simulink model "signal_control_system"  (R2023a)
settings: Solver=FixedStepDiscrete  StartTime=0.0  StopTime=20  FixedStep=1  RelTol=1e-3
settings Model: Creator=Administrator  LastModifiedBy=Administrator
settings DataIOCC: ExternalInput=[t, ia, ib, ic, Tlevel, PClimit, set_val, PC, FC]  LoadExternalInput=on  SaveFormat=Structure  ReturnWorkspaceOutputs=off

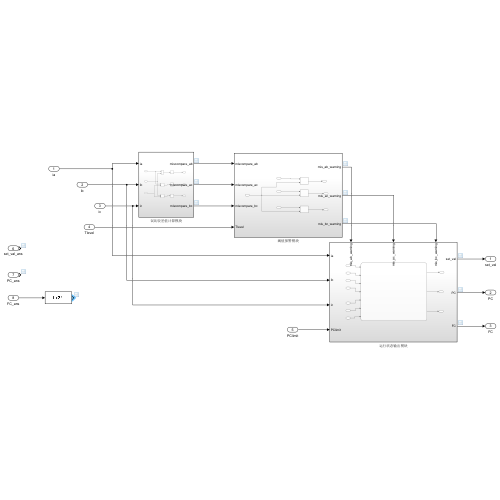
[thumbnail: Simulink's stored preview of the top-level diagram]
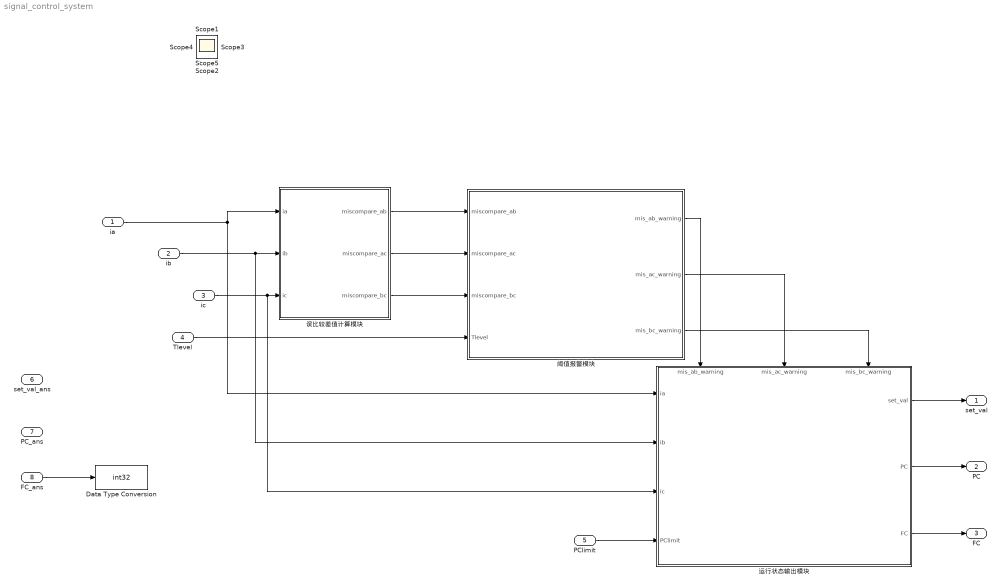
== system signal_control_system ==
  ia : Inport  PortDimensions=1
  ib : Inport  Port=2  PortDimensions=1
  ic : Inport  Port=3  PortDimensions=1
  Tlevel : Inport  Port=4  PortDimensions=1
  PClimit : Inport  Port=5  OutDataTypeStr=double  PortDimensions=1
  set_val_ans : Inport  Port=6
  PC_ans : Inport  Port=7
  FC_ans : Inport  Port=8  OutDataTypeStr=double
  Data Type Conversion : DataTypeConversion  OutDataTypeStr=int32  SaturateOnIntegerOverflow=off  RndMeth=Floor
  误比较差值计算模块 : Subsystem
  运行状态输出模块 : Subsystem
      settings: PortSchema="{\"entries\":[{\"content\":{\"sides\":[{\"content\":{\"connectorIds\":[\"In1\",\"In2\",\"In3\",\"In4\"]},\"type\":\"ConnectorPlacement.EquallySpacedRectSide\",\"uuid\":\"c2265341-80b0-436b-af31-29986e0e6bdd\"},{\"content\":{\"connectorIds\":[\"Out1\",\"Out2\",\"Out3\"],\"side\":\"RIGHT\"},\"type\":\"ConnectorPlacement.EquallySpacedRectSide\",\"uuid\":\"b242c194-baa4-408e-b219-ab790b6c0c89\"},{\"content\":{\"connectorIds\":[\"In5\",\"In6\",\"In7\"],\"side\":\"TOP\"},\"type\":\"ConnectorPlacement.EquallySpacedRectSide\",\"uuid\":\"72118fcd-d084-4d5a-ad77-022196fa3641\"}]},\"type\":\"ConnectorPlacement.EquallySpacedConnector\",\"uuid\":\"1dca4bdc-c94a-404e-99f4-c038544fbae3\"}],\"packageUris\":[\"http://schema.mathworks.com/mf0/Connector/R2020b\"],\"version\":\"1.0\"}"
  阈值报警模块 : Subsystem
  set_val : Outport
  PC : Outport  Port=2
  FC : Outport  Port=3
  Scope{,1..5} (6 alike) : Scope
  wires:
  ia/1 -> 运行状态输出模块/1(ia), 误比较差值计算模块/1(ia)
  ib/1 -> 运行状态输出模块/2(ib), 误比较差值计算模块/2(ib)
  ic/1 -> 误比较差值计算模块/3(ic), 运行状态输出模块/3(ic)
  误比较差值计算模块/1(miscompare_ab) -> 阈值报警模块/1(miscompare_ab)
  误比较差值计算模块/2(miscompare_ac) -> 阈值报警模块/2(miscompare_ac)
  误比较差值计算模块/3(miscompare_bc) -> 阈值报警模块/3(miscompare_bc)
  Tlevel/1 -> 阈值报警模块/4(Tlevel)
  阈值报警模块/1(mis_ab_warning) -> 运行状态输出模块/5(mis_ab_warning)
  阈值报警模块/2(mis_ac_warning) -> 运行状态输出模块/6(mis_ac_warning)
  阈值报警模块/3(mis_bc_warning) -> 运行状态输出模块/7(mis_bc_warning)
  运行状态输出模块/1(set_val) -> set_val/1
  运行状态输出模块/2(PC) -> PC/1
  运行状态输出模块/3(FC) -> FC/1
  PClimit/1 -> 运行状态输出模块/4(PClimit)
  FC_ans/1 -> Data Type Conversion/1

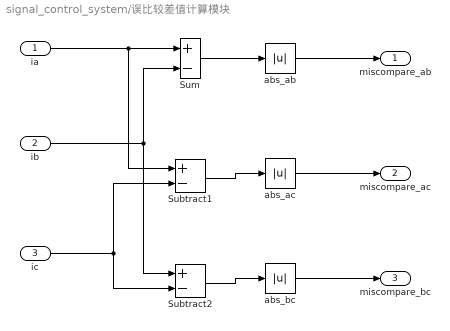
== system signal_control_system/误比较差值计算模块 ==
  ia : Inport
  ib : Inport  Port=2
  ic : Inport  Port=3
  Subtract1 : Sum  Inputs=+-
  Subtract2 : Sum  Inputs=+-
  Sum : Sum  Inputs=+-
  abs_ab : Abs  SaturateOnIntegerOverflow=off
  abs_ac : Abs  SaturateOnIntegerOverflow=off
  abs_bc : Abs  SaturateOnIntegerOverflow=off
  miscompare_ab : Outport
  miscompare_ac : Outport  Port=2
  miscompare_bc : Outport  Port=3
  wires:
  ia/1 -> Subtract1/1, Sum/1
  Subtract1/1 -> abs_ac/1
  abs_bc/1 -> miscompare_bc/1
  abs_ac/1 -> miscompare_ac/1
  Sum/1 -> abs_ab/1
  Subtract2/1 -> abs_bc/1
  abs_ab/1 -> miscompare_ab/1
  ic/1 -> Subtract2/2, Subtract1/2
  ib/1 -> Sum/2, Subtract2/1

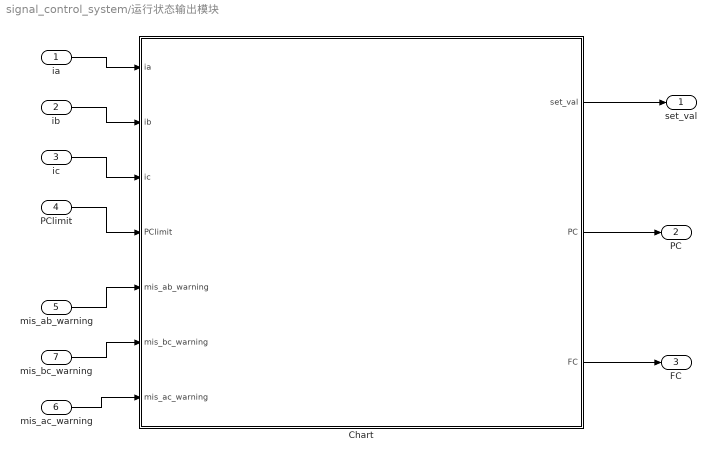
== system signal_control_system/运行状态输出模块 ==
  ia : Inport
  ib : Inport  Port=2
  ic : Inport  Port=3
  PClimit : Inport  Port=4
  mis_ab_warning : Inport  Port=5  OutDataTypeStr=boolean
  mis_ac_warning : Inport  Port=6  OutDataTypeStr=boolean
  mis_bc_warning : Inport  Port=7  OutDataTypeStr=boolean
  Chart : Stateflow chart  TreatAsAtomicUnit=on
  set_val : Outport
  PC : Outport  Port=2
  FC : Outport  Port=3
  wires:
  ia/1 -> Chart/1(ia)
  ib/1 -> Chart/2(ib)
  ic/1 -> Chart/3(ic)
  PClimit/1 -> Chart/4(PClimit)
  mis_ab_warning/1 -> Chart/5(mis_ab_warning)
  mis_bc_warning/1 -> Chart/6(mis_bc_warning)
  mis_ac_warning/1 -> Chart/7(mis_ac_warning)
  Chart/1(set_val) -> set_val/1
  Chart/2(PC) -> PC/1
  Chart/3(FC) -> FC/1

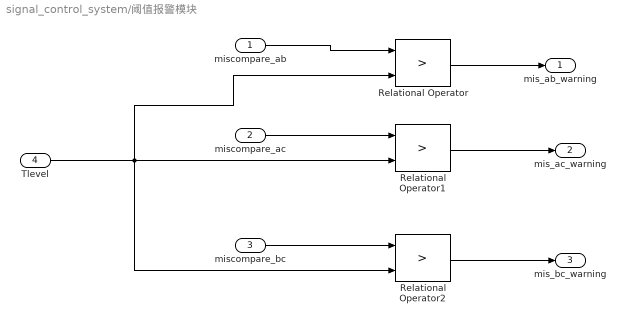
== system signal_control_system/阈值报警模块 ==
  miscompare_ab : Inport
  miscompare_ac : Inport  Port=2
  miscompare_bc : Inport  Port=3
  Tlevel : Inport  Port=4
  Relational Operator : RelationalOperator  Operator=>  OutDataTypeStr=boolean  RndMeth=Simplest
  Relational Operator1 : RelationalOperator  Operator=>  OutDataTypeStr=boolean  RndMeth=Simplest
  Relational Operator2 : RelationalOperator  Operator=>  OutDataTypeStr=boolean  RndMeth=Simplest
  mis_ab_warning : Outport  OutDataTypeStr=boolean
  mis_ac_warning : Outport  Port=2  OutDataTypeStr=boolean
  mis_bc_warning : Outport  Port=3  OutDataTypeStr=boolean
  wires:
  Tlevel/1 -> Relational Operator/2, Relational Operator2/2, Relational Operator1/2
  Relational Operator1/1 -> mis_ac_warning/1
  miscompare_ac/1 -> Relational Operator1/1
  Relational Operator2/1 -> mis_bc_warning/1
  Relational Operator/1 -> mis_ab_warning/1
  miscompare_ab/1 -> Relational Operator/1
  miscompare_bc/1 -> Relational Operator2/1

== stateflow chart signal_control_system/运行状态输出模块/Chart ==
  state SingleFault_ia
    entry:
    FC = 1;
    PC = 0;
    set_val = (ib + ic) / 2;
    during:
    set_val = (ib + ic) / 2;
    if (mis_ab_warning && mis_ac_warning && mis_bc_warning)
    PC = PC + 1;
    end
  state NoFault
    entry:
    FC = 0;
    PC = 0;
    set_val  = median([ia, ib, ic]);
    during:
    set_val  = median([ia, ib, ic]);
    if (~mis_ab_warning && ~mis_ac_warning && ~mis_bc_warning)
    PC = PC ;
    else
    PC = PC + 1;
    end
  state MultiFault
    entry:
    FC = -1;
    PC = 0;
  state SingleFault_ib
    entry:
    FC = 2;
    PC = 0;
    set_val = (ia + ic) / 2;
    during:
    set_val = (ia + ic) / 2;
    if (mis_ab_warning && mis_ac_warning && mis_bc_warning)
    PC = PC + 1;
    end
  state SingleFault_ic
    entry:
    FC = 4;
    PC = 0;
    set_val = (ib + ia) / 2;
    during:
    set_val = (ib + ia) / 2;
    if (mis_ab_warning && mis_ac_warning && mis_bc_warning)
    PC = PC + 1;
    end
  NoFault -> SingleFault_ia [order 1] : [mis_ab_warning && mis_ac_warning && ~mis_bc_warning && PC > PClimit]
  SingleFault_ia -> MultiFault [order 1] : [mis_ab_warning && mis_ac_warning && mis_bc_warning && PC > PClimit]
  SingleFault_ia -> NoFault [order 2] : [~mis_ab_warning && ~mis_ac_warning && ~mis_bc_warning]
  (default) -> NoFault
  SingleFault_ib -> MultiFault [order 1] : [mis_ab_warning && mis_ac_warning && mis_bc_warning && PC > PClimit]
  SingleFault_ib -> NoFault [order 2] : [~mis_ab_warning && ~mis_ac_warning && ~mis_bc_warning]
  NoFault -> SingleFault_ib [order 2] : [mis_ab_warning && ~mis_ac_warning && mis_bc_warning && PC > PClimit]
  NoFault -> MultiFault [order 4] : [mis_ab_warning && mis_ac_warning && mis_bc_warning && PC > PClimit ]
  SingleFault_ic -> MultiFault [order 1] : [mis_ab_warning && mis_ac_warning && mis_bc_warning && PC > PClimit]
  NoFault -> SingleFault_ic [order 3] : [~mis_ab_warning && mis_ac_warning && mis_bc_warning && PC > PClimit]
  SingleFault_ic -> NoFault [order 2] : [~mis_ab_warning && ~mis_ac_warning && ~mis_bc_warning]
  data: ia input double; ib input double; ic input double; PClimit input double; set_val output double; PC output int32; FC output int32; mis_ab_warning input boolean; mis_bc_warning input boolean; mis_ac_warning input boolean
